simulink model "TokenRing10Node"  (R2022a)
settings: Solver=VariableStepAuto  StartTime=0.0  StopTime=1000  RelTol=1e-3
undefined symbols (not defined in the file): m, n
settings Model: SimulationMode=accelerator  Creator=aurisb  LastModifiedBy=aurisb

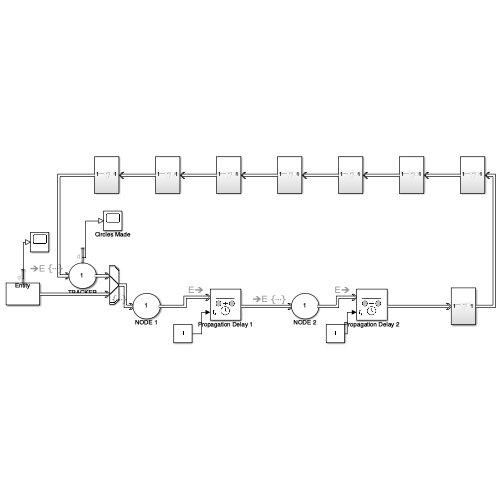
[thumbnail: Simulink's stored preview of the top-level diagram]
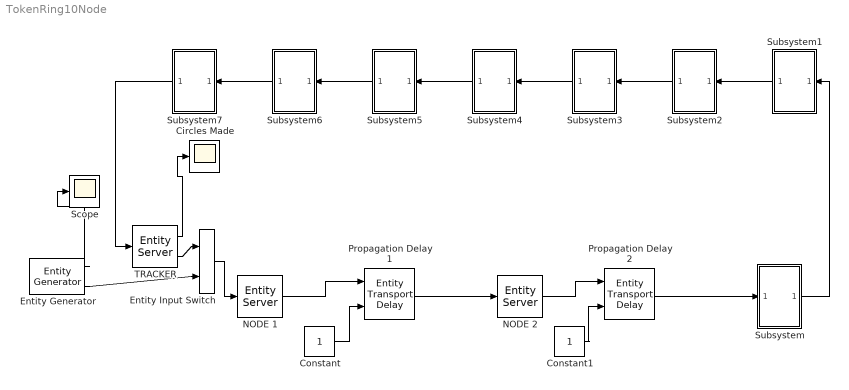
== system TokenRing10Node ==
  Circles Made : Scope
  Constant : Constant
  Constant1 : Constant
  Entity Input Switch : EntityInputSwitch  InputPortMessageModes=m,m  OutputPortMessageModes=m
  Entity Generator : EntityGenerator  OutputPortMessageModes=n,m  Period=inf  AttributeName=token|ACK|Source|Destination|ServiceTimeValue|FrameSize|data|totalPasses|usefulPasses  AttributeInitialValue=0|0|1|1|0|4472|1|0|1  NumberEntitiesDeparted=on  EntityType=Structured  EntityTypeName=Entity
      settings: OutputPortMap=o0,o3
  NODE 1 : EntityServer  InputPortMessageModes=m  OutputPortMessageModes=m  Capacity=1  ServiceTimeSource=Attribute  ServiceTimeValue=5  ServiceTimeAttributeName=ServiceTimeValue  EntryAction=|
      | myid = 1;
      | totalNodes = 10;
      | persistent dataToSend;
      | if isempty(dataToSend)
      | 	dataToSend = 17888;
      | end
      | 
      | entity.totalPasses = entity.totalPasses+1;
      | 
      | %If token is an ACK meant for you, free it 
      | if entity.ACK == 1
      | 	if entity.Destination == myid %CHANGE
      | 		entity.usefulPasses = entity.usefulPasses+1;
      | 		disp("Node " + myid + " received ACK from " + entity.Source + ". Releasing free token.");
      | 		entity.ACK=0;
      | 		entity.token=0;
      |     else
      |     	disp("Node " + myid + " passing along ACK to " + entity.Destination + ".");
      |     end
      | end
      |     
      | 
      | %If token is not free token
      | if entity.token == 1
      | 	%if it is meant for you
      | 	if entity.Destination == myid %CHANGE
      | 		entity.usefulPasses = entity.usefulPasses+1;
      | 		disp("Node " + myid + " received data, sending ACK back to " + entity.Source);
      | 
      | 		%if it is meant for you as an ACK, free it
      | 		if entity.ACK==1
      | 			entity.ACK=0;
      | 			entity.token=0;
      | 		%if it is meant for you as a message, send back an ACK
      | 		else
      | 			entity.ACK=1;
      | 			entity.Destination = entity.Source;
      | 			entity.Source=myid; %CHANGE
      | 	    end
      | 
      | 	%if it is meant for someone else, pass it on
      | 	else
      | 		disp("Node " + myid + " passing along token from " + entity.Source + " to " + entity.Destination + ".");
      | 		%do nothing and pass it on
      | 	end
      | end
      | 
      | %If it it is a free token, send data
      | if entity.token == 0 && dataToSend > 0
      | 
      | 	entity.token=1;
      | 	destinationPossibilities = setdiff(1:totalNodes, myid);
      | 	entity.Destination = destinationPossibilities(ceil(numel(destinationPossibilities) * rand));
      | 	
      | 	%entity.Destination = randi([1,totalNodes-1]);
      | 	%if entity.Destination == myid
      | 	%		entity.Destination = anotherid;
      | 	%end
      | 	entity.Source=myid; %CHANGE
      | 	dataToSend = dataToSend-4472;
      | 	entity.data=4472;
      | 	disp("Node "+myid+ " sending 4472 bytes of data to " + entity.Destination+ ". Node 1 has " + dataToSend + " bytes of data remaining to send.");
      | else if entity.token == 0
      | 	disp("Node " + myid + " has no data to send, passing token along.");
      | end
  NODE 2 : EntityServer  InputPortMessageModes=m  OutputPortMessageModes=m  Capacity=1  ServiceTimeSource=Attribute  ServiceTimeValue=5  ServiceTimeAttributeName=ServiceTimeValue  EntryAction=|
      | myid = 2;
      | totalNodes = 10;
      | persistent dataToSend;
      | if isempty(dataToSend)
      | 	dataToSend = 17888;
      | end
      | 
      | entity.totalPasses = entity.totalPasses+1;
      | 
      | %If token is an ACK meant for you, free it 
      | if entity.ACK == 1
      | 	if entity.Destination == myid %CHANGE
      | 		entity.usefulPasses = entity.usefulPasses+1;
      | 		disp("Node " + myid + " received ACK from " + entity.Source + ". Releasing free token.");
      | 		entity.ACK=0;
      | 		entity.token=0;
      |     else
      |     	disp("Node " + myid + " passing along ACK to " + entity.Destination + ".");
      |     end
      | end
      |     
      | 
      | %If token is not free token
      | if entity.token == 1
      | 	%if it is meant for you
      | 	if entity.Destination == myid %CHANGE
      | 		entity.usefulPasses = entity.usefulPasses+1;
      | 		disp("Node " + myid + " received data, sending ACK back to " + entity.Source);
      | 
      | 		%if it is meant for you as an ACK, free it
      | 		if entity.ACK==1
      | 			entity.ACK=0;
      | 			entity.token=0;
      | 		%if it is meant for you as a message, send back an ACK
      | 		else
      | 			entity.ACK=1;
      | 			entity.Destination = entity.Source;
      | 			entity.Source=myid; %CHANGE
      | 	    end
      | 
      | 	%if it is meant for someone else, pass it on
      | 	else
      | 		disp("Node " + myid + " passing along token from " + entity.Source + " to " + entity.Destination + ".");
      | 		%do nothing and pass it on
      | 	end
      | end
      | 
      | %If it it is a free token, send data
      | if entity.token == 0 && dataToSend > 0
      | 
      | 	entity.token=1;
      | 	destinationPossibilities = setdiff(1:totalNodes, myid);
      | 	entity.Destination = destinationPossibilities(ceil(numel(destinationPossibilities) * rand));
      | 	
      | 	%entity.Destination = randi([1,totalNodes-1]);
      | 	%if entity.Destination == myid
      | 	%		entity.Destination = anotherid;
      | 	%end
      | 	entity.Source=myid; %CHANGE
      | 	dataToSend = dataToSend-4472;
      | 	entity.data=4472;
      | 	disp("Node "+myid+ " sending 4472 bytes of data to " + entity.Destination+ ". Node 1 has " + dataToSend + " bytes of data remaining to send.");
      | else if entity.token == 0
      | 	disp("Node " + myid + " has no data to send, passing token along.");
      | end
  Propagation Delay 1 : EntityTransportDelay  InputPortMessageModes=m,n  OutputPortMessageModes=m
  Propagation Delay 2 : EntityTransportDelay  InputPortMessageModes=m,n  OutputPortMessageModes=m
  Scope : Scope
  Subsystem : Subsystem
  Subsystem1 : Subsystem
  Subsystem2 : Subsystem
  Subsystem3 : Subsystem
  Subsystem4 : Subsystem
  Subsystem5 : Subsystem
  Subsystem6 : Subsystem
  Subsystem7 : Subsystem
  TRACKER : EntityServer  InputPortMessageModes=m  OutputPortMessageModes=n,m  Capacity=1  ServiceTimeValue=0  EntryAction=|  NumberEntitiesDeparted=on
      | persistent loops;
      | if isempty(loops)
      | 	loops = 0;
      | end
      | loops = loops + 1;
      | coder.extrinsic('get_param');
      | disp(get_param('TokenRing10Node','SimulationTime'));
      | disp("[TRACKER] Loops done around ring: " + loops + ".");
      | disp("[TRACKER] Total Passes: " + entity.totalPasses + ". Useful Passes: " + entity.usefulPasses + ".");
      settings: OutputPortMap=o0,o9
  wires:
  NODE 2/1 -> Propagation Delay 2/1
  Entity Generator/2 -> Entity Input Switch/2
  Entity Input Switch/1 -> NODE 1/1
  Entity Generator/1 -> Scope/1
  TRACKER/2 -> Entity Input Switch/1
  TRACKER/1 -> Circles Made/1
  NODE 1/1 -> Propagation Delay 1/1
  Propagation Delay 1/1 -> NODE 2/1
  Constant/1 -> Propagation Delay 1/2
  Constant1/1 -> Propagation Delay 2/2
  Propagation Delay 2/1 -> Subsystem/1(In1)
  Subsystem3/1(Out1) -> Subsystem4/1(In1)
  Subsystem6/1(Out1) -> Subsystem7/1(In1)
  Subsystem/1(Out1) -> Subsystem1/1(In1)
  Subsystem1/1(Out1) -> Subsystem2/1(In1)
  Subsystem2/1(Out1) -> Subsystem3/1(In1)
  Subsystem4/1(Out1) -> Subsystem5/1(In1)
  Subsystem5/1(Out1) -> Subsystem6/1(In1)
  Subsystem7/1(Out1) -> TRACKER/1

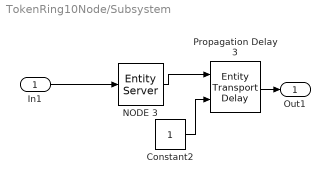
== system TokenRing10Node/Subsystem ==
  In1 : Inport
  Constant2 : Constant
  NODE 3 : EntityServer  InputPortMessageModes=m  OutputPortMessageModes=m  Capacity=1  ServiceTimeSource=Attribute  ServiceTimeValue=5  ServiceTimeAttributeName=ServiceTimeValue  EntryAction=|
      | myid = 3;
      | totalNodes = 10;
      | persistent dataToSend;
      | if isempty(dataToSend)
      | 	dataToSend = 17888;
      | end
      | 
      | entity.totalPasses = entity.totalPasses+1;
      | 
      | %If token is an ACK meant for you, free it 
      | if entity.ACK == 1
      | 	if entity.Destination == myid %CHANGE
      | 		entity.usefulPasses = entity.usefulPasses+1;
      | 		disp("Node " + myid + " received ACK from " + entity.Source + ". Releasing free token.");
      | 		entity.ACK=0;
      | 		entity.token=0;
      |     else
      |     	disp("Node " + myid + " passing along ACK to " + entity.Destination + ".");
      |     end
      | end
      |     
      | 
      | %If token is not free token
      | if entity.token == 1
      | 	%if it is meant for you
      | 	if entity.Destination == myid %CHANGE
      | 		entity.usefulPasses = entity.usefulPasses+1;
      | 		disp("Node " + myid + " received data, sending ACK back to " + entity.Source);
      | 
      | 		%if it is meant for you as an ACK, free it
      | 		if entity.ACK==1
      | 			entity.ACK=0;
      | 			entity.token=0;
      | 		%if it is meant for you as a message, send back an ACK
      | 		else
      | 			entity.ACK=1;
      | 			entity.Destination = entity.Source;
      | 			entity.Source=myid; %CHANGE
      | 	    end
      | 
      | 	%if it is meant for someone else, pass it on
      | 	else
      | 		disp("Node " + myid + " passing along token from " + entity.Source + " to " + entity.Destination + ".");
      | 		%do nothing and pass it on
      | 	end
      | end
      | 
      | %If it it is a free token, send data
      | if entity.token == 0 && dataToSend > 0
      | 
      | 	entity.token=1;
      | 	destinationPossibilities = setdiff(1:totalNodes, myid);
      | 	entity.Destination = destinationPossibilities(ceil(numel(destinationPossibilities) * rand));
      | 	
      | 	%entity.Destination = randi([1,totalNodes-1]);
      | 	%if entity.Destination == myid
      | 	%		entity.Destination = anotherid;
      | 	%end
      | 	entity.Source=myid; %CHANGE
      | 	dataToSend = dataToSend-4472;
      | 	entity.data=4472;
      | 	disp("Node "+myid+ " sending 4472 bytes of data to " + entity.Destination+ ". Node 1 has " + dataToSend + " bytes of data remaining to send.");
      | else if entity.token == 0
      | 	disp("Node " + myid + " has no data to send, passing token along.");
      | end
  Propagation Delay 3 : EntityTransportDelay  InputPortMessageModes=m,n  OutputPortMessageModes=m
  Out1 : Outport
  wires:
  Constant2/1 -> Propagation Delay 3/2
  In1/1 -> NODE 3/1
  Propagation Delay 3/1 -> Out1/1
  NODE 3/1 -> Propagation Delay 3/1

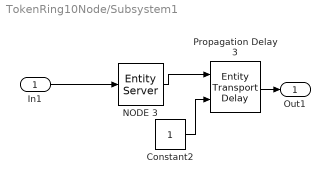
== system TokenRing10Node/Subsystem1 ==
  In1 : Inport
  Constant2 : Constant
  NODE 3 : EntityServer  InputPortMessageModes=m  OutputPortMessageModes=m  Capacity=1  ServiceTimeSource=Attribute  ServiceTimeValue=5  ServiceTimeAttributeName=ServiceTimeValue  EntryAction=|
      | myid = 4;
      | totalNodes = 10;
      | persistent dataToSend;
      | if isempty(dataToSend)
      | 	dataToSend = 17888;
      | end
      | 
      | entity.totalPasses = entity.totalPasses+1;
      | 
      | %If token is an ACK meant for you, free it 
      | if entity.ACK == 1
      | 	if entity.Destination == myid %CHANGE
      | 		entity.usefulPasses = entity.usefulPasses+1;
      | 		disp("Node " + myid + " received ACK from " + entity.Source + ". Releasing free token.");
      | 		entity.ACK=0;
      | 		entity.token=0;
      |     else
      |     	disp("Node " + myid + " passing along ACK to " + entity.Destination + ".");
      |     end
      | end
      |     
      | 
      | %If token is not free token
      | if entity.token == 1
      | 	%if it is meant for you
      | 	if entity.Destination == myid %CHANGE
      | 		entity.usefulPasses = entity.usefulPasses+1;
      | 		disp("Node " + myid + " received data, sending ACK back to " + entity.Source);
      | 
      | 		%if it is meant for you as an ACK, free it
      | 		if entity.ACK==1
      | 			entity.ACK=0;
      | 			entity.token=0;
      | 		%if it is meant for you as a message, send back an ACK
      | 		else
      | 			entity.ACK=1;
      | 			entity.Destination = entity.Source;
      | 			entity.Source=myid; %CHANGE
      | 	    end
      | 
      | 	%if it is meant for someone else, pass it on
      | 	else
      | 		disp("Node " + myid + " passing along token from " + entity.Source + " to " + entity.Destination + ".");
      | 		%do nothing and pass it on
      | 	end
      | end
      | 
      | %If it it is a free token, send data
      | if entity.token == 0 && dataToSend > 0
      | 
      | 	entity.token=1;
      | 	destinationPossibilities = setdiff(1:totalNodes, myid);
      | 	entity.Destination = destinationPossibilities(ceil(numel(destinationPossibilities) * rand));
      | 	
      | 	%entity.Destination = randi([1,totalNodes-1]);
      | 	%if entity.Destination == myid
      | 	%		entity.Destination = anotherid;
      | 	%end
      | 	entity.Source=myid; %CHANGE
      | 	dataToSend = dataToSend-4472;
      | 	entity.data=4472;
      | 	disp("Node "+myid+ " sending 4472 bytes of data to " + entity.Destination+ ". Node 1 has " + dataToSend + " bytes of data remaining to send.");
      | else if entity.token == 0
      | 	disp("Node " + myid + " has no data to send, passing token along.");
      | end
  Propagation Delay 3 : EntityTransportDelay  InputPortMessageModes=m,n  OutputPortMessageModes=m
  Out1 : Outport
  wires:
  Constant2/1 -> Propagation Delay 3/2
  In1/1 -> NODE 3/1
  Propagation Delay 3/1 -> Out1/1
  NODE 3/1 -> Propagation Delay 3/1

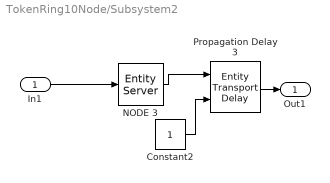
== system TokenRing10Node/Subsystem2 ==
  In1 : Inport
  Constant2 : Constant
  NODE 3 : EntityServer  InputPortMessageModes=m  OutputPortMessageModes=m  Capacity=1  ServiceTimeSource=Attribute  ServiceTimeValue=5  ServiceTimeAttributeName=ServiceTimeValue  EntryAction=|
      | myid = 5;
      | totalNodes = 10;
      | persistent dataToSend;
      | if isempty(dataToSend)
      | 	dataToSend = 17888;
      | end
      | 
      | entity.totalPasses = entity.totalPasses+1;
      | 
      | %If token is an ACK meant for you, free it 
      | if entity.ACK == 1
      | 	if entity.Destination == myid %CHANGE
      | 		entity.usefulPasses = entity.usefulPasses+1;
      | 		disp("Node " + myid + " received ACK from " + entity.Source + ". Releasing free token.");
      | 		entity.ACK=0;
      | 		entity.token=0;
      |     else
      |     	disp("Node " + myid + " passing along ACK to " + entity.Destination + ".");
      |     end
      | end
      |     
      | 
      | %If token is not free token
      | if entity.token == 1
      | 	%if it is meant for you
      | 	if entity.Destination == myid %CHANGE
      | 		entity.usefulPasses = entity.usefulPasses+1;
      | 		disp("Node " + myid + " received data, sending ACK back to " + entity.Source);
      | 
      | 		%if it is meant for you as an ACK, free it
      | 		if entity.ACK==1
      | 			entity.ACK=0;
      | 			entity.token=0;
      | 		%if it is meant for you as a message, send back an ACK
      | 		else
      | 			entity.ACK=1;
      | 			entity.Destination = entity.Source;
      | 			entity.Source=myid; %CHANGE
      | 	    end
      | 
      | 	%if it is meant for someone else, pass it on
      | 	else
      | 		disp("Node " + myid + " passing along token from " + entity.Source + " to " + entity.Destination + ".");
      | 		%do nothing and pass it on
      | 	end
      | end
      | 
      | %If it it is a free token, send data
      | if entity.token == 0 && dataToSend > 0
      | 
      | 	entity.token=1;
      | 	destinationPossibilities = setdiff(1:totalNodes, myid);
      | 	entity.Destination = destinationPossibilities(ceil(numel(destinationPossibilities) * rand));
      | 	
      | 	%entity.Destination = randi([1,totalNodes-1]);
      | 	%if entity.Destination == myid
      | 	%		entity.Destination = anotherid;
      | 	%end
      | 	entity.Source=myid; %CHANGE
      | 	dataToSend = dataToSend-4472;
      | 	entity.data=4472;
      | 	disp("Node "+myid+ " sending 4472 bytes of data to " + entity.Destination+ ". Node 1 has " + dataToSend + " bytes of data remaining to send.");
      | else if entity.token == 0
      | 	disp("Node " + myid + " has no data to send, passing token along.");
      | end
  Propagation Delay 3 : EntityTransportDelay  InputPortMessageModes=m,n  OutputPortMessageModes=m
  Out1 : Outport
  wires:
  Constant2/1 -> Propagation Delay 3/2
  In1/1 -> NODE 3/1
  Propagation Delay 3/1 -> Out1/1
  NODE 3/1 -> Propagation Delay 3/1

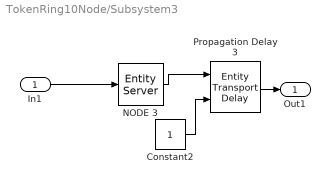
== system TokenRing10Node/Subsystem3 ==
  In1 : Inport
  Constant2 : Constant
  NODE 3 : EntityServer  InputPortMessageModes=m  OutputPortMessageModes=m  Capacity=1  ServiceTimeSource=Attribute  ServiceTimeValue=5  ServiceTimeAttributeName=ServiceTimeValue  EntryAction=|
      | myid = 6;
      | totalNodes = 10;
      | persistent dataToSend;
      | if isempty(dataToSend)
      | 	dataToSend = 17888;
      | end
      | 
      | entity.totalPasses = entity.totalPasses+1;
      | 
      | %If token is an ACK meant for you, free it 
      | if entity.ACK == 1
      | 	if entity.Destination == myid %CHANGE
      | 		entity.usefulPasses = entity.usefulPasses+1;
      | 		disp("Node " + myid + " received ACK from " + entity.Source + ". Releasing free token.");
      | 		entity.ACK=0;
      | 		entity.token=0;
      |     else
      |     	disp("Node " + myid + " passing along ACK to " + entity.Destination + ".");
      |     end
      | end
      |     
      | 
      | %If token is not free token
      | if entity.token == 1
      | 	%if it is meant for you
      | 	if entity.Destination == myid %CHANGE
      | 		entity.usefulPasses = entity.usefulPasses+1;
      | 		disp("Node " + myid + " received data, sending ACK back to " + entity.Source);
      | 
      | 		%if it is meant for you as an ACK, free it
      | 		if entity.ACK==1
      | 			entity.ACK=0;
      | 			entity.token=0;
      | 		%if it is meant for you as a message, send back an ACK
      | 		else
      | 			entity.ACK=1;
      | 			entity.Destination = entity.Source;
      | 			entity.Source=myid; %CHANGE
      | 	    end
      | 
      | 	%if it is meant for someone else, pass it on
      | 	else
      | 		disp("Node " + myid + " passing along token from " + entity.Source + " to " + entity.Destination + ".");
      | 		%do nothing and pass it on
      | 	end
      | end
      | 
      | %If it it is a free token, send data
      | if entity.token == 0 && dataToSend > 0
      | 
      | 	entity.token=1;
      | 	destinationPossibilities = setdiff(1:totalNodes, myid);
      | 	entity.Destination = destinationPossibilities(ceil(numel(destinationPossibilities) * rand));
      | 	
      | 	%entity.Destination = randi([1,totalNodes-1]);
      | 	%if entity.Destination == myid
      | 	%		entity.Destination = anotherid;
      | 	%end
      | 	entity.Source=myid; %CHANGE
      | 	dataToSend = dataToSend-4472;
      | 	entity.data=4472;
      | 	disp("Node "+myid+ " sending 4472 bytes of data to " + entity.Destination+ ". Node 1 has " + dataToSend + " bytes of data remaining to send.");
      | else if entity.token == 0
      | 	disp("Node " + myid + " has no data to send, passing token along.");
      | end
  Propagation Delay 3 : EntityTransportDelay  InputPortMessageModes=m,n  OutputPortMessageModes=m
  Out1 : Outport
  wires:
  Constant2/1 -> Propagation Delay 3/2
  In1/1 -> NODE 3/1
  Propagation Delay 3/1 -> Out1/1
  NODE 3/1 -> Propagation Delay 3/1

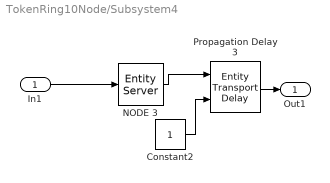
== system TokenRing10Node/Subsystem4 ==
  In1 : Inport
  Constant2 : Constant
  NODE 3 : EntityServer  InputPortMessageModes=m  OutputPortMessageModes=m  Capacity=1  ServiceTimeSource=Attribute  ServiceTimeValue=5  ServiceTimeAttributeName=ServiceTimeValue  EntryAction=|
      | myid = 7;
      | totalNodes = 10;
      | persistent dataToSend;
      | if isempty(dataToSend)
      | 	dataToSend = 17888;
      | end
      | 
      | entity.totalPasses = entity.totalPasses+1;
      | 
      | %If token is an ACK meant for you, free it 
      | if entity.ACK == 1
      | 	if entity.Destination == myid %CHANGE
      | 		entity.usefulPasses = entity.usefulPasses+1;
      | 		disp("Node " + myid + " received ACK from " + entity.Source + ". Releasing free token.");
      | 		entity.ACK=0;
      | 		entity.token=0;
      |     else
      |     	disp("Node " + myid + " passing along ACK to " + entity.Destination + ".");
      |     end
      | end
      |     
      | 
      | %If token is not free token
      | if entity.token == 1
      | 	%if it is meant for you
      | 	if entity.Destination == myid %CHANGE
      | 		entity.usefulPasses = entity.usefulPasses+1;
      | 		disp("Node " + myid + " received data, sending ACK back to " + entity.Source);
      | 
      | 		%if it is meant for you as an ACK, free it
      | 		if entity.ACK==1
      | 			entity.ACK=0;
      | 			entity.token=0;
      | 		%if it is meant for you as a message, send back an ACK
      | 		else
      | 			entity.ACK=1;
      | 			entity.Destination = entity.Source;
      | 			entity.Source=myid; %CHANGE
      | 	    end
      | 
      | 	%if it is meant for someone else, pass it on
      | 	else
      | 		disp("Node " + myid + " passing along token from " + entity.Source + " to " + entity.Destination + ".");
      | 		%do nothing and pass it on
      | 	end
      | end
      | 
      | %If it it is a free token, send data
      | if entity.token == 0 && dataToSend > 0
      | 
      | 	entity.token=1;
      | 	destinationPossibilities = setdiff(1:totalNodes, myid);
      | 	entity.Destination = destinationPossibilities(ceil(numel(destinationPossibilities) * rand));
      | 	
      | 	%entity.Destination = randi([1,totalNodes-1]);
      | 	%if entity.Destination == myid
      | 	%		entity.Destination = anotherid;
      | 	%end
      | 	entity.Source=myid; %CHANGE
      | 	dataToSend = dataToSend-4472;
      | 	entity.data=4472;
      | 	disp("Node "+myid+ " sending 4472 bytes of data to " + entity.Destination+ ". Node 1 has " + dataToSend + " bytes of data remaining to send.");
      | else if entity.token == 0
      | 	disp("Node " + myid + " has no data to send, passing token along.");
      | end
  Propagation Delay 3 : EntityTransportDelay  InputPortMessageModes=m,n  OutputPortMessageModes=m
  Out1 : Outport
  wires:
  Constant2/1 -> Propagation Delay 3/2
  In1/1 -> NODE 3/1
  Propagation Delay 3/1 -> Out1/1
  NODE 3/1 -> Propagation Delay 3/1

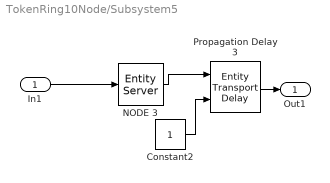
== system TokenRing10Node/Subsystem5 ==
  In1 : Inport
  Constant2 : Constant
  NODE 3 : EntityServer  InputPortMessageModes=m  OutputPortMessageModes=m  Capacity=1  ServiceTimeSource=Attribute  ServiceTimeValue=5  ServiceTimeAttributeName=ServiceTimeValue  EntryAction=|
      | myid = 8;
      | totalNodes = 10;
      | persistent dataToSend;
      | if isempty(dataToSend)
      | 	dataToSend = 17888;
      | end
      | 
      | entity.totalPasses = entity.totalPasses+1;
      | 
      | %If token is an ACK meant for you, free it 
      | if entity.ACK == 1
      | 	if entity.Destination == myid %CHANGE
      | 		entity.usefulPasses = entity.usefulPasses+1;
      | 		disp("Node " + myid + " received ACK from " + entity.Source + ". Releasing free token.");
      | 		entity.ACK=0;
      | 		entity.token=0;
      |     else
      |     	disp("Node " + myid + " passing along ACK to " + entity.Destination + ".");
      |     end
      | end
      |     
      | 
      | %If token is not free token
      | if entity.token == 1
      | 	%if it is meant for you
      | 	if entity.Destination == myid %CHANGE
      | 		entity.usefulPasses = entity.usefulPasses+1;
      | 		disp("Node " + myid + " received data, sending ACK back to " + entity.Source);
      | 
      | 		%if it is meant for you as an ACK, free it
      | 		if entity.ACK==1
      | 			entity.ACK=0;
      | 			entity.token=0;
      | 		%if it is meant for you as a message, send back an ACK
      | 		else
      | 			entity.ACK=1;
      | 			entity.Destination = entity.Source;
      | 			entity.Source=myid; %CHANGE
      | 	    end
      | 
      | 	%if it is meant for someone else, pass it on
      | 	else
      | 		disp("Node " + myid + " passing along token from " + entity.Source + " to " + entity.Destination + ".");
      | 		%do nothing and pass it on
      | 	end
      | end
      | 
      | %If it it is a free token, send data
      | if entity.token == 0 && dataToSend > 0
      | 
      | 	entity.token=1;
      | 	destinationPossibilities = setdiff(1:totalNodes, myid);
      | 	entity.Destination = destinationPossibilities(ceil(numel(destinationPossibilities) * rand));
      | 	
      | 	%entity.Destination = randi([1,totalNodes-1]);
      | 	%if entity.Destination == myid
      | 	%		entity.Destination = anotherid;
      | 	%end
      | 	entity.Source=myid; %CHANGE
      | 	dataToSend = dataToSend-4472;
      | 	entity.data=4472;
      | 	disp("Node "+myid+ " sending 4472 bytes of data to " + entity.Destination+ ". Node 1 has " + dataToSend + " bytes of data remaining to send.");
      | else if entity.token == 0
      | 	disp("Node " + myid + " has no data to send, passing token along.");
      | end
  Propagation Delay 3 : EntityTransportDelay  InputPortMessageModes=m,n  OutputPortMessageModes=m
  Out1 : Outport
  wires:
  Constant2/1 -> Propagation Delay 3/2
  In1/1 -> NODE 3/1
  Propagation Delay 3/1 -> Out1/1
  NODE 3/1 -> Propagation Delay 3/1

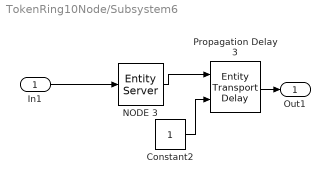
== system TokenRing10Node/Subsystem6 ==
  In1 : Inport
  Constant2 : Constant
  NODE 3 : EntityServer  InputPortMessageModes=m  OutputPortMessageModes=m  Capacity=1  ServiceTimeSource=Attribute  ServiceTimeValue=5  ServiceTimeAttributeName=ServiceTimeValue  EntryAction=|
      | myid = 9;
      | totalNodes = 10;
      | persistent dataToSend;
      | if isempty(dataToSend)
      | 	dataToSend = 17888;
      | end
      | 
      | entity.totalPasses = entity.totalPasses+1;
      | 
      | %If token is an ACK meant for you, free it 
      | if entity.ACK == 1
      | 	if entity.Destination == myid %CHANGE
      | 		entity.usefulPasses = entity.usefulPasses+1;
      | 		disp("Node " + myid + " received ACK from " + entity.Source + ". Releasing free token.");
      | 		entity.ACK=0;
      | 		entity.token=0;
      |     else
      |     	disp("Node " + myid + " passing along ACK to " + entity.Destination + ".");
      |     end
      | end
      |     
      | 
      | %If token is not free token
      | if entity.token == 1
      | 	%if it is meant for you
      | 	if entity.Destination == myid %CHANGE
      | 		entity.usefulPasses = entity.usefulPasses+1;
      | 		disp("Node " + myid + " received data, sending ACK back to " + entity.Source);
      | 
      | 		%if it is meant for you as an ACK, free it
      | 		if entity.ACK==1
      | 			entity.ACK=0;
      | 			entity.token=0;
      | 		%if it is meant for you as a message, send back an ACK
      | 		else
      | 			entity.ACK=1;
      | 			entity.Destination = entity.Source;
      | 			entity.Source=myid; %CHANGE
      | 	    end
      | 
      | 	%if it is meant for someone else, pass it on
      | 	else
      | 		disp("Node " + myid + " passing along token from " + entity.Source + " to " + entity.Destination + ".");
      | 		%do nothing and pass it on
      | 	end
      | end
      | 
      | %If it it is a free token, send data
      | if entity.token == 0 && dataToSend > 0
      | 
      | 	entity.token=1;
      | 	destinationPossibilities = setdiff(1:totalNodes, myid);
      | 	entity.Destination = destinationPossibilities(ceil(numel(destinationPossibilities) * rand));
      | 	
      | 	%entity.Destination = randi([1,totalNodes-1]);
      | 	%if entity.Destination == myid
      | 	%		entity.Destination = anotherid;
      | 	%end
      | 	entity.Source=myid; %CHANGE
      | 	dataToSend = dataToSend-4472;
      | 	entity.data=4472;
      | 	disp("Node "+myid+ " sending 4472 bytes of data to " + entity.Destination+ ". Node 1 has " + dataToSend + " bytes of data remaining to send.");
      | else if entity.token == 0
      | 	disp("Node " + myid + " has no data to send, passing token along.");
      | end
  Propagation Delay 3 : EntityTransportDelay  InputPortMessageModes=m,n  OutputPortMessageModes=m
  Out1 : Outport
  wires:
  Constant2/1 -> Propagation Delay 3/2
  In1/1 -> NODE 3/1
  Propagation Delay 3/1 -> Out1/1
  NODE 3/1 -> Propagation Delay 3/1

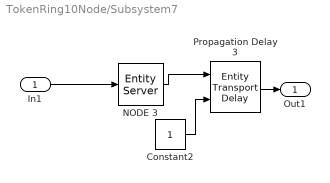
== system TokenRing10Node/Subsystem7 ==
  In1 : Inport
  Constant2 : Constant
  NODE 3 : EntityServer  InputPortMessageModes=m  OutputPortMessageModes=m  Capacity=1  ServiceTimeSource=Attribute  ServiceTimeValue=5  ServiceTimeAttributeName=ServiceTimeValue  EntryAction=|
      | myid = 10;
      | totalNodes = 10;
      | persistent dataToSend;
      | if isempty(dataToSend)
      | 	dataToSend = 17888;
      | end
      | 
      | entity.totalPasses = entity.totalPasses+1;
      | 
      | %If token is an ACK meant for you, free it 
      | if entity.ACK == 1
      | 	if entity.Destination == myid %CHANGE
      | 		entity.usefulPasses = entity.usefulPasses+1;
      | 		disp("Node " + myid + " received ACK from " + entity.Source + ". Releasing free token.");
      | 		entity.ACK=0;
      | 		entity.token=0;
      |     else
      |     	disp("Node " + myid + " passing along ACK to " + entity.Destination + ".");
      |     end
      | end
      |     
      | 
      | %If token is not free token
      | if entity.token == 1
      | 	%if it is meant for you
      | 	if entity.Destination == myid %CHANGE
      | 		entity.usefulPasses = entity.usefulPasses+1;
      | 		disp("Node " + myid + " received data, sending ACK back to " + entity.Source);
      | 
      | 		%if it is meant for you as an ACK, free it
      | 		if entity.ACK==1
      | 			entity.ACK=0;
      | 			entity.token=0;
      | 		%if it is meant for you as a message, send back an ACK
      | 		else
      | 			entity.ACK=1;
      | 			entity.Destination = entity.Source;
      | 			entity.Source=myid; %CHANGE
      | 	    end
      | 
      | 	%if it is meant for someone else, pass it on
      | 	else
      | 		disp("Node " + myid + " passing along token from " + entity.Source + " to " + entity.Destination + ".");
      | 		%do nothing and pass it on
      | 	end
      | end
      | 
      | %If it it is a free token, send data
      | if entity.token == 0 && dataToSend > 0
      | 
      | 	entity.token=1;
      | 	destinationPossibilities = setdiff(1:totalNodes, myid);
      | 	entity.Destination = destinationPossibilities(ceil(numel(destinationPossibilities) * rand));
      | 	
      | 	%entity.Destination = randi([1,totalNodes-1]);
      | 	%if entity.Destination == myid
      | 	%		entity.Destination = anotherid;
      | 	%end
      | 	entity.Source=myid; %CHANGE
      | 	dataToSend = dataToSend-4472;
      | 	entity.data=4472;
      | 	disp("Node "+myid+ " sending 4472 bytes of data to " + entity.Destination+ ". Node 1 has " + dataToSend + " bytes of data remaining to send.");
      | else if entity.token == 0
      | 	disp("Node " + myid + " has no data to send, passing token along.");
      | end
  Propagation Delay 3 : EntityTransportDelay  InputPortMessageModes=m,n  OutputPortMessageModes=m
  Out1 : Outport
  wires:
  Constant2/1 -> Propagation Delay 3/2
  In1/1 -> NODE 3/1
  Propagation Delay 3/1 -> Out1/1
  NODE 3/1 -> Propagation Delay 3/1
